simulink model "HydroEye_6DOF_OpenLoop"  (R2024b)
settings: Solver=VariableStepAuto  StartTime=0.0  StopTime=120  RelTol=1e-3
undefined symbols (not defined in the file or in its folder): b, c, CD, cg, CL, Cl, Clp, Clr, Cm, Cmq, Cn, Cnp, Cnr, cp, CY, Earth, mass, WGS84
libraries: simulink_extras x4, aerolibasang x2, shared6dof x1, aerolibatmos2 x1, aerolibadyn x1, aerolibtransform2 x1
settings Model: Creator=01  LastModifiedBy=01
settings OptimizationCC: ReuseModelBlockBuffer=off
settings RTWCC: GPUComputeCapability=3.5

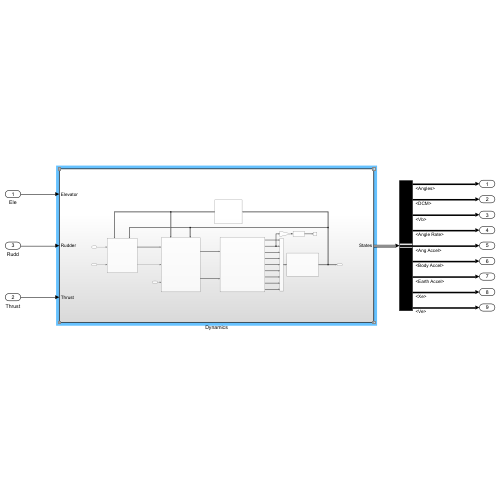
[thumbnail: Simulink's stored preview of the top-level diagram]
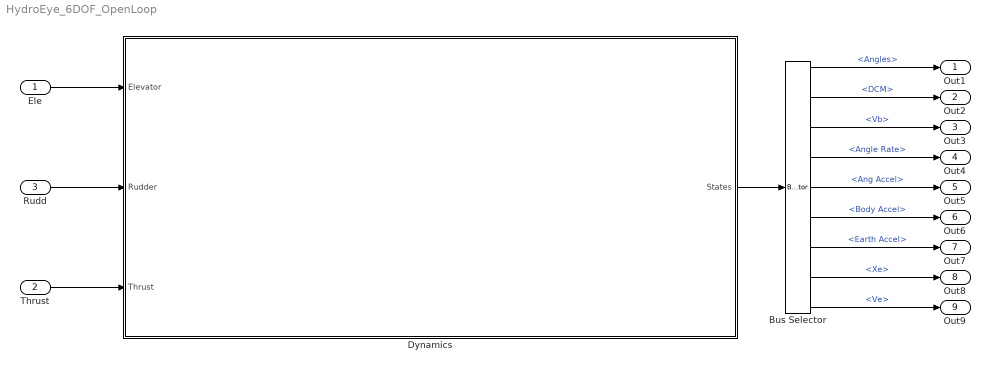
== system HydroEye_6DOF_OpenLoop ==
  Ele : Inport
  Thrust : Inport  Port=2
  Rudd : Inport  Port=3
  Bus Selector : BusSelector  OutputSignals=Raw States.Angles,Raw States.DCM,Raw States.Vb,Raw States.Angle Rate,Raw States.Ang Accel,Raw States.Body Accel,Raw States.Earth Accel,Raw States.Xe,Raw States.Ve
  Dynamics : Subsystem
  Out1 : Outport
  Out2 : Outport  Port=2
  Out3 : Outport  Port=3
  Out4 : Outport  Port=4
  Out5 : Outport  Port=5
  Out6 : Outport  Port=6
  Out7 : Outport  Port=7
  Out8 : Outport  Port=8
  Out9 : Outport  Port=9
  wires:
  Ele/1 -> Dynamics/1(Elevator)
  Thrust/1 -> Dynamics/3(Thrust)
  Dynamics/1(States) -> Bus Selector/1
  Bus Selector/1 -> Out1/1  "<Angles>"
  Bus Selector/2 -> Out2/1  "<DCM>"
  Bus Selector/3 -> Out3/1  "<Vb>"
  Bus Selector/4 -> Out4/1  "<Angle Rate>"
  Bus Selector/5 -> Out5/1  "<Ang Accel>"
  Bus Selector/6 -> Out6/1  "<Body Accel>"
  Bus Selector/7 -> Out7/1  "<Earth Accel>"
  Bus Selector/8 -> Out8/1  "<Xe>"
  Bus Selector/9 -> Out9/1  "<Ve>"
  Rudd/1 -> Dynamics/2(Rudder)

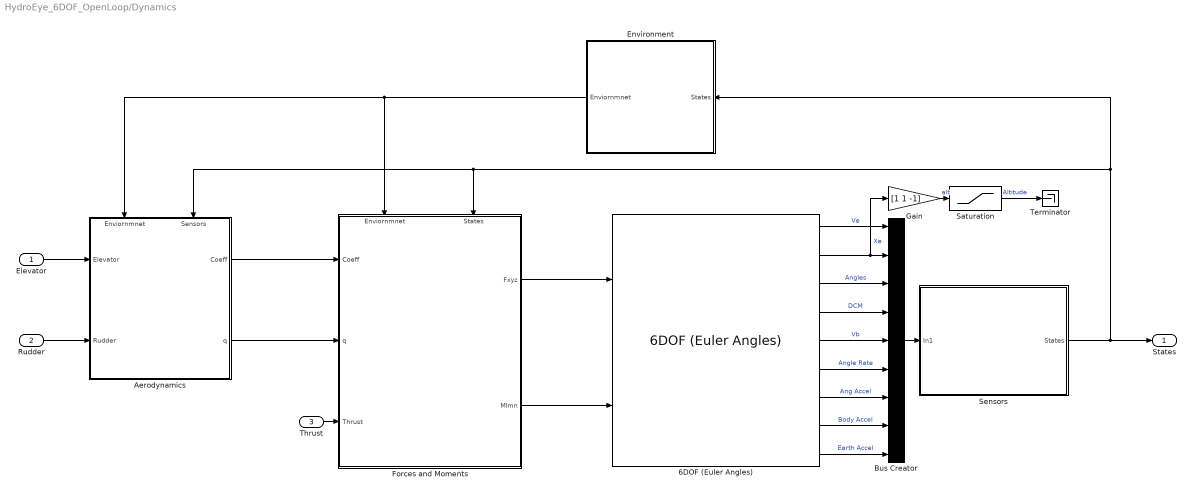
== system HydroEye_6DOF_OpenLoop/Dynamics ==
  Elevator : Inport
  Rudder : Inport  Port=2
  Thrust : Inport  Port=3
  6DOF (Euler Angles) : shared6dof/6DOF (Euler Angles)  units=Metric (MKS)  mtype=Fixed  rep=Euler Angles  xme_0=init.pos  Vm_0=init.v  eul_0=[ 0 deg2rad(2.4) 0 ]  pm_0=[ 0 0 0 ]  mass_0=mass  mass_e=0.5  mass_f=2.0  inertia=I  inertia_e=eye(3)  inertia_f=2*eye(3)  k_quat=1.0  vre_flag=on  abi_flag=on  aMode=aMode  xme_statename=''  Vm_statename=''  eul_statename=''  quat_statename=''  pm_statename=''  mass_statename=''
      settings: LibrarySourceBlock=|
      | aeroblk_lib_HL20/HL20
      | Airframe/6DOF (Euler Angles)
  Aerodynamics : Subsystem
      settings: PortSchema="{\"entries\":[{\"content\":{\"sides\":[{\"content\":{\"connectorIds\":[\"In1\",\"In2\"]},\"type\":\"ConnectorPlacement.EquallySpacedRectSide\",\"uuid\":\"6872a9e6-04cc-43fe-8307-2d3d33caa71d\"},{\"content\":{\"side\":\"RIGHT\"},\"type\":\"ConnectorPlacement.EquallySpacedRectSide\",\"uuid\":\"de5f8d1c-5c0e-46cb-94c5-3e4cce4cf93c\"},{\"content\":{\"connectorIds\":[\"In3\",\"In4\"],\"side\":\"TOP\"},\"type\":\"ConnectorPlacement.EquallySpacedRectSide\",\"uuid\":\"d9dd98e0-8ff1-4387-90e5-0ec057a718ca\"},{\"content\":{\"connectorIds\":[\"Out1\",\"Out2\"],\"side\":\"BOTTOM\"},\"type\":\"ConnectorPlacement.EquallySpacedRectSide\",\"uuid\":\"12421dae-0177-4f1a-9b31-64f8981b692b\"}]},\"type\":\"ConnectorPlacement.EquallySpacedConnector\",\"uuid\":\"9e39648a-6fb6-4479-b0ac-1c0f654141e6\"}],\"packageUris\":[\"http://schema.mathworks.com/mf0/Connector/R2020b\"],\"version\":\"1.0\"}"
  Bus Creator : BusCreator  Inputs=9
  "Environment " : Subsystem
      settings: LibrarySourceBlock=|
      | aeroblk_lib_HL20/HL20
      | Airframe/Environment Models
  Forces and Moments : Subsystem
      settings: PortSchema="{\"entries\":[{\"content\":{\"sides\":[{\"content\":{\"connectorIds\":[\"In1\",\"In2\",\"In3\"]},\"type\":\"ConnectorPlacement.EquallySpacedRectSide\",\"uuid\":\"3fce203a-ae0b-4bce-a87b-30de4173aaf5\"},{\"content\":{\"connectorIds\":[\"Out1\",\"Out2\"],\"side\":\"RIGHT\"},\"type\":\"ConnectorPlacement.EquallySpacedRectSide\",\"uuid\":\"d2fe57eb-25a4-4a3f-81a0-5ad8de127e30\"},{\"content\":{\"connectorIds\":[\"In4\",\"In5\"],\"side\":\"TOP\"},\"type\":\"ConnectorPlacement.EquallySpacedRectSide\",\"uuid\":\"a48e6f39-78f9-49f0-a87f-61fc55168fed\"}]},\"type\":\"ConnectorPlacement.EquallySpacedConnector\",\"uuid\":\"9bf99150-9e27-4a02-9f3a-86824a85a991\"}],\"packageUris\":[\"http://schema.mathworks.com/mf0/Connector/R2020b\"],\"version\":\"1.0\"}"
      settings: LibrarySourceBlock=|
      | aeroblk_lib_HL20/HL20
      | Airframe/Forces and Moments
  Gain : Gain  Gain=[1 1 -1]
  Saturation : Saturate  UpperLimit=inf  LowerLimit=0
  Sensors : Subsystem
  Terminator : Terminator
  States : Outport
  wires:
  6DOF (Euler Angles)/6 -> Bus Creator/6  "Angle Rate"
  6DOF (Euler Angles)/5 -> Bus Creator/5  "Vb"
  Aerodynamics/1(Coeff) -> Forces and Moments/1(Coeff)
  6DOF (Euler Angles)/9 -> Bus Creator/9  "Earth Accel"
  Gain/1 -> Saturation/1  "alt"
  Aerodynamics/2(q) -> Forces and Moments/2(q)
  6DOF (Euler Angles)/1 -> Bus Creator/1  "Ve"
  6DOF (Euler Angles)/3 -> Bus Creator/3  "Angles"
  6DOF (Euler Angles)/7 -> Bus Creator/7  "Ang Accel"
  6DOF (Euler Angles)/4 -> Bus Creator/4  "DCM"
  Bus Creator/1 -> Sensors/1(In1)
  "Environment "/1(Enviornmnet) -> Forces and Moments/4(Enviornmnet), Aerodynamics/1(Enviornmnet)
  Forces and Moments/2(Mlmn) -> 6DOF (Euler Angles)/2
  Forces and Moments/1(Fxyz) -> 6DOF (Euler Angles)/1
  Saturation/1 -> Terminator/1  "Altitude"
  Sensors/1(States) -> "Environment "/1(States), Aerodynamics/2(Sensors), Forces and Moments/5(States), States/1
  6DOF (Euler Angles)/2 -> Gain/1, Bus Creator/2  "Xe"
  6DOF (Euler Angles)/8 -> Bus Creator/8  "Body Accel"
  Elevator/1 -> Aerodynamics/3(Elevator)
  Thrust/1 -> Forces and Moments/3(Thrust)
  Rudder/1 -> Aerodynamics/4(Rudder)

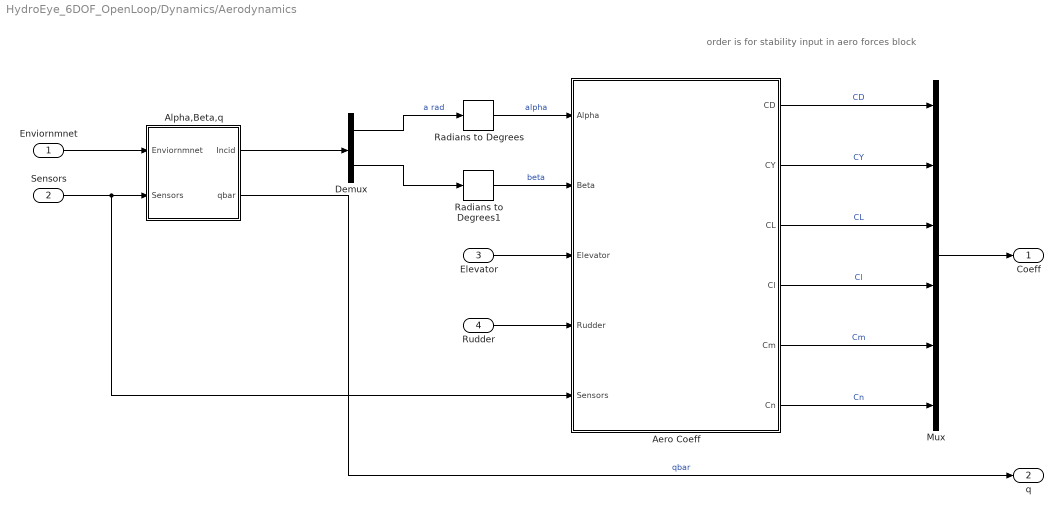
== system HydroEye_6DOF_OpenLoop/Dynamics/Aerodynamics ==
  note: order is for stability input in aero forces block
  Enviornmnet : Inport
  Sensors : Inport  Port=2
  Elevator : Inport  Port=3
  Rudder : Inport  Port=4
  Aero Coeff : Subsystem
  Alpha,Beta,q : Subsystem
      settings: LibrarySourceBlock=|
      | aeroblk_lib_HL20/HL20
      | Airframe/Alpha,Beta,Mach
  Demux : Demux  Outputs=2
  Mux : Mux  Inputs=6
  Radians to Degrees : simulink_extras/Transformations/Radians to Degrees
  Radians to Degrees1 : simulink_extras/Transformations/Radians to Degrees
  Coeff : Outport
  q : Outport  Port=2
  wires:
  Sensors/1 -> Aero Coeff/5(Sensors), Alpha,Beta,q/2(Sensors)
  Enviornmnet/1 -> Alpha,Beta,q/1(Enviornmnet)
  Alpha,Beta,q/2(qbar) -> q/1  "qbar"
  Mux/1 -> Coeff/1
  Alpha,Beta,q/1(Incid) -> Demux/1
  Aero Coeff/1(CD) -> Mux/1  "CD"
  Aero Coeff/2(CY) -> Mux/2  "CY"
  Aero Coeff/3(CL) -> Mux/3  "CL"
  Aero Coeff/4(Cl) -> Mux/4  "Cl"
  Aero Coeff/5(Cm) -> Mux/5  "Cm"
  Aero Coeff/6(Cn) -> Mux/6  "Cn"
  Radians to Degrees/1 -> Aero Coeff/1(Alpha)  "alpha"
  Radians to Degrees1/1 -> Aero Coeff/2(Beta)  "beta"
  Demux/2 -> Radians to Degrees1/1
  Demux/1 -> Radians to Degrees/1  "a rad"
  Elevator/1 -> Aero Coeff/3(Elevator)
  Rudder/1 -> Aero Coeff/4(Rudder)

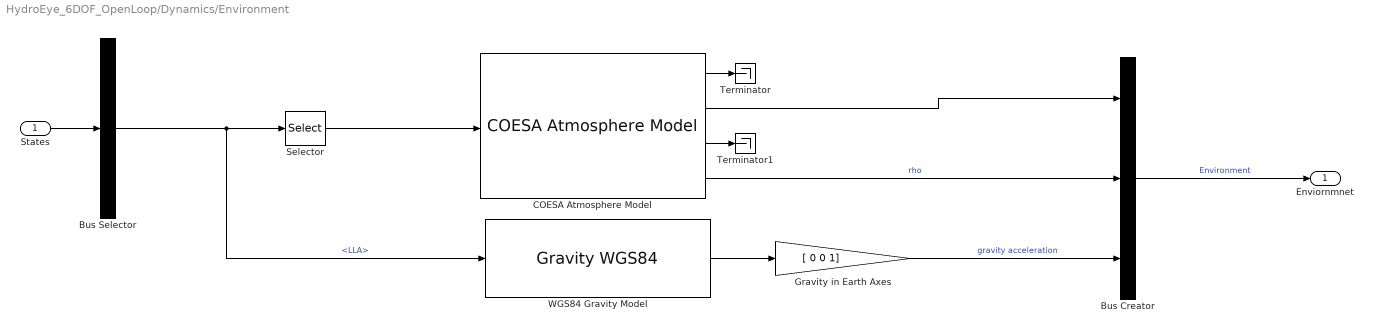
== system HydroEye_6DOF_OpenLoop/Dynamics/Environment  ==
  States : Inport
  Bus Creator : BusCreator  Inputs=3
  Bus Selector : BusSelector  OutputSignals=LLA
  COESA Atmosphere Model : aerolibatmos2/COESA Atmosphere Model  units=Metric (MKS)  spec=1976 COESA-extended U.S. Standard Atmosphere  model=Profile  profile_var=High temperature  profile_percent=10%  profile_alt=5 km (16404 ft)  envelope_var=High temperature  envelope_percent=1%  action=None
      settings: LibrarySourceBlock=|
      | aeroblk_lib_HL20/HL20
      | Airframe/Environment Models/COESA Atmosphere Model
  Gravity in Earth Axes : Gain  Gain=[ 0 0 1]  SaturateOnIntegerOverflow=on  OutDataTypeStr=Inherit: Same as input  ParamDataTypeStr=Inherit: Same as input
  Selector : Selector  InputPortWidth=3  IndexOptions=Index vector (dialog)  Indices=3  OutputSizes=1
  Terminator : Terminator
  Terminator1 : Terminator
  "WGS84 Gravity Model  " : GravityWGS84  action=None
  Enviornmnet : Outport
  wires:
  "WGS84 Gravity Model  "/1 -> Gravity in Earth Axes/1
  COESA Atmosphere Model/1 -> Terminator/1
  COESA Atmosphere Model/3 -> Terminator1/1
  COESA Atmosphere Model/2 -> Bus Creator/1
  COESA Atmosphere Model/4 -> Bus Creator/2  "rho"
  Selector/1 -> COESA Atmosphere Model/1
  Gravity in Earth Axes/1 -> Bus Creator/3  "gravity acceleration"
  States/1 -> Bus Selector/1
  Bus Selector/1 -> "WGS84 Gravity Model  "/1, Selector/1  "<LLA>"
  Bus Creator/1 -> Enviornmnet/1  "Environment"

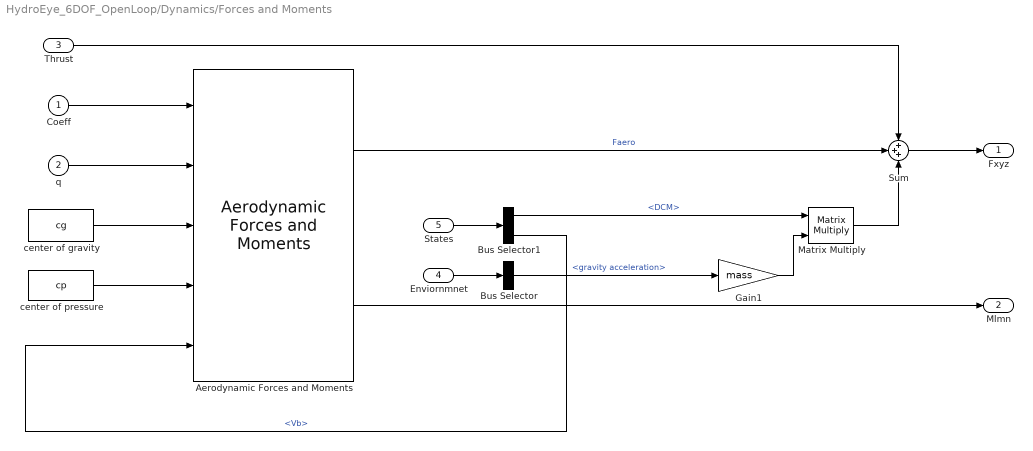
== system HydroEye_6DOF_OpenLoop/Dynamics/Forces and Moments ==
  Coeff : Inport
  q : Inport  Port=2  Unit=Pa
  Thrust : Inport  Port=3
  Enviornmnet : Inport  Port=4
  States : Inport  Port=5
  Aerodynamic Forces and Moments : aerolibadyn/Aerodynamic Forces and Moments   inputAxes=Stability  outputForceAxes=Body  outputMomentAxes=Body  S=Sref  b=b  cbar=c
      settings: LibrarySourceBlock=|
      | aeroblk_lib_HL20/HL20
      | Airframe/Forces and Moments/Aerodynamic
      | Forces and Moments
  Bus Selector : BusSelector  OutputSignals=gravity acceleration
  Bus Selector1 : BusSelector  OutputSignals=Raw States.DCM,Raw States.Vb
  Gain1 : Gain  Gain=mass
  Matrix Multiply : Product  Multiplication=Matrix(*)
  Sum : Sum  Inputs=+++  InputSameDT=on  SaturateOnIntegerOverflow=on  OutDataTypeStr=Inherit: Same as first input
  center of gravity : Constant  Value=cg
  center of pressure : Constant  Value=cp
  Fxyz : Outport
  Mlmn : Outport  Port=2
  wires:
  Coeff/1 -> Aerodynamic Forces and Moments/1
  q/1 -> Aerodynamic Forces and Moments/2
  Sum/1 -> Fxyz/1
  center of gravity/1 -> Aerodynamic Forces and Moments/3
  center of pressure/1 -> Aerodynamic Forces and Moments/4
  Enviornmnet/1 -> Bus Selector/1
  States/1 -> Bus Selector1/1
  Matrix Multiply/1 -> Sum/3
  Bus Selector/1 -> Gain1/1  "<gravity acceleration>"
  Gain1/1 -> Matrix Multiply/2
  Bus Selector1/1 -> Matrix Multiply/1  "<DCM>"
  Thrust/1 -> Sum/1
  Aerodynamic Forces and Moments/1 -> Sum/2  "Faero"
  Aerodynamic Forces and Moments/2 -> Mlmn/1
  Bus Selector1/2 -> Aerodynamic Forces and Moments/5  "<Vb>"

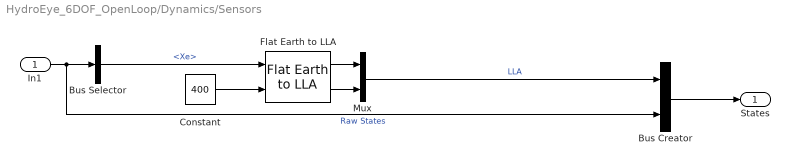
== system HydroEye_6DOF_OpenLoop/Dynamics/Sensors ==
  In1 : Inport
  Bus Creator : BusCreator  Inputs=2
  Bus Selector : BusSelector  OutputSignals=Xe
  Constant : Constant  Value=400
  Flat Earth to LLA : aerolibtransform2/Flat Earth to LLA  units=Metric (MKS)  ptype=Earth (WGS84)  F=1/298.257223563  R=6378137  refPosPort=off  LL0=[ 24 46 ]  psi=0
  Mux : Mux  Inputs=2
  States : Outport
  wires:
  In1/1 -> Bus Creator/2, Bus Selector/1  "Raw States"
  Bus Selector/1 -> Flat Earth to LLA/1  "<Xe>"
  Flat Earth to LLA/2 -> Mux/2
  Flat Earth to LLA/1 -> Mux/1
  Mux/1 -> Bus Creator/1  "LLA"
  Bus Creator/1 -> States/1
  Constant/1 -> Flat Earth to LLA/2

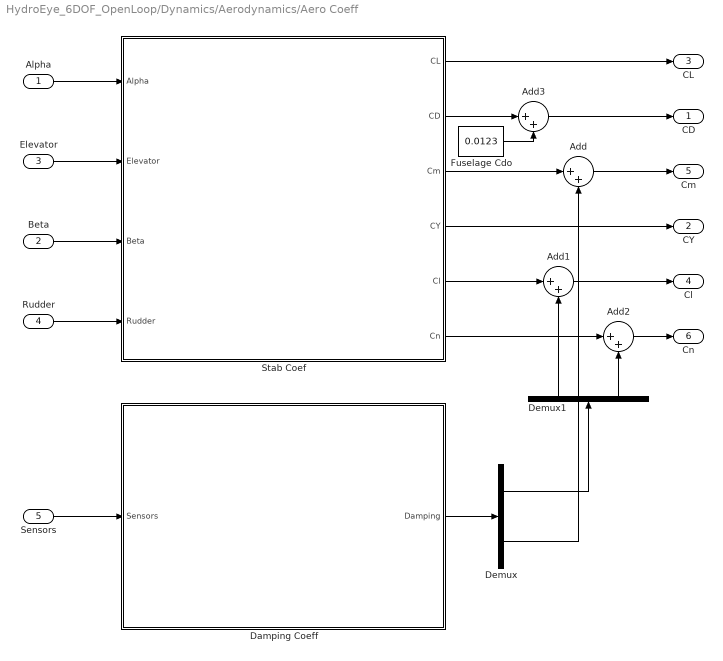
== system HydroEye_6DOF_OpenLoop/Dynamics/Aerodynamics/Aero Coeff ==
  Alpha : Inport
  Beta : Inport  Port=2
  Elevator : Inport  Port=3
  Rudder : Inport  Port=4
  Sensors : Inport  Port=5
  Add{,1..3} (4 alike) : Sum  Inputs=|++
  Damping Coeff : Subsystem
  Demux : Demux  Outputs=2
  Demux1 : Demux  Outputs=2
  Fuselage Cdo : Constant  Value=0.0123
  Stab Coef : Subsystem
  CD : Outport
  CY : Outport  Port=2
  CL : Outport  Port=3
  Cl : Outport  Port=4
  Cm : Outport  Port=5
  Cn : Outport  Port=6
  wires:
  Alpha/1 -> Stab Coef/1(Alpha)
  Elevator/1 -> Stab Coef/2(Elevator)
  Beta/1 -> Stab Coef/3(Beta)
  Rudder/1 -> Stab Coef/4(Rudder)
  Stab Coef/1(CL) -> CL/1
  Stab Coef/4(CY) -> CY/1
  Sensors/1 -> Damping Coeff/1(Sensors)
  Damping Coeff/1(Damping) -> Demux/1
  Stab Coef/3(Cm) -> Add/1
  Add/1 -> Cm/1
  Demux/2 -> Add/2
  Stab Coef/5(Cl) -> Add1/1
  Add1/1 -> Cl/1
  Add2/1 -> Cn/1
  Stab Coef/6(Cn) -> Add2/1
  Demux/1 -> Demux1/1
  Demux1/2 -> Add2/2
  Demux1/1 -> Add1/2
  Stab Coef/2(CD) -> Add3/1
  Add3/1 -> CD/1
  Fuselage Cdo/1 -> Add3/2

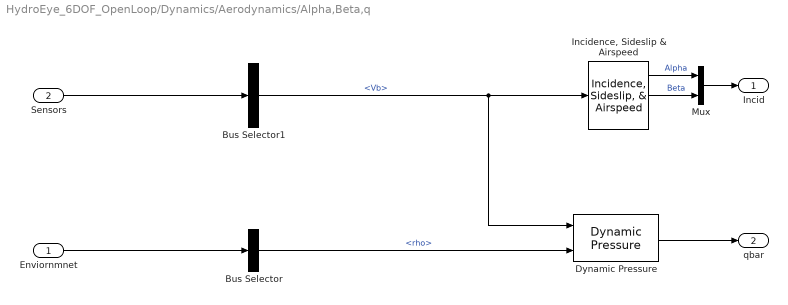
== system HydroEye_6DOF_OpenLoop/Dynamics/Aerodynamics/Alpha,Beta,q ==
  Enviornmnet : Inport
  Sensors : Inport  Port=2
  Bus Selector : BusSelector  OutputSignals=rho
  Bus Selector1 : BusSelector  OutputSignals=Raw States.Vb
  Dynamic Pressure : aerolibasang/Dynamic Pressure
      settings: LibrarySourceBlock=|
      | aeroblk_lib_HL20/HL20
      | Airframe/Alpha,Beta,Mach/Dynamic Pressure
  "Incidence, Sideslip & Airspeed" : aerolibasang/Incidence, Sideslip, & Airspeed
      settings: LibrarySourceBlock=|
      | aeroblk_lib_HL20/HL20
      | Airframe/Alpha,Beta,Mach/Incidence, Sideslip
      | & Airspeed
  Mux : Mux  Inputs=2
  Incid : Outport  Unit=rad  VectorParamsAs1DForOutWhenUnconnected=off
  qbar : Outport  Port=2  Unit=Pa  InitialOutput=0  VectorParamsAs1DForOutWhenUnconnected=off
  wires:
  "Incidence, Sideslip & Airspeed"/1 -> Mux/1  "Alpha"
  Mux/1 -> Incid/1
  "Incidence, Sideslip & Airspeed"/2 -> Mux/2  "Beta"
  Dynamic Pressure/1 -> qbar/1
  Enviornmnet/1 -> Bus Selector/1
  Bus Selector/1 -> Dynamic Pressure/2  "<rho>"
  Sensors/1 -> Bus Selector1/1
  Bus Selector1/1 -> "Incidence, Sideslip & Airspeed"/1, Dynamic Pressure/1  "<Vb>"

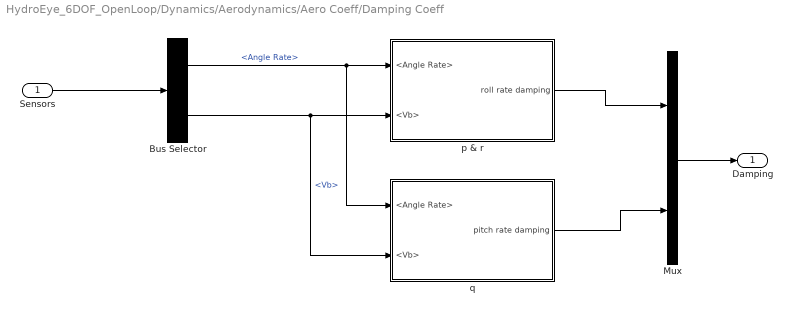
== system HydroEye_6DOF_OpenLoop/Dynamics/Aerodynamics/Aero Coeff/Damping Coeff ==
  Sensors : Inport
  Bus Selector : BusSelector  OutputSignals=Raw States.Angle Rate,Raw States.Vb
  Mux : Mux  Inputs=2
  p & r : Subsystem
  q : Subsystem
  Damping : Outport
  wires:
  Sensors/1 -> Bus Selector/1
  q/1(pitch rate damping) -> Mux/2
  Mux/1 -> Damping/1
  p & r/1(roll rate damping) -> Mux/1
  Bus Selector/1 -> q/1(<Angle Rate>), p & r/1(<Angle Rate>)  "<Angle Rate>"
  Bus Selector/2 -> q/2(<Vb>), p & r/2(<Vb>)  "<Vb>"

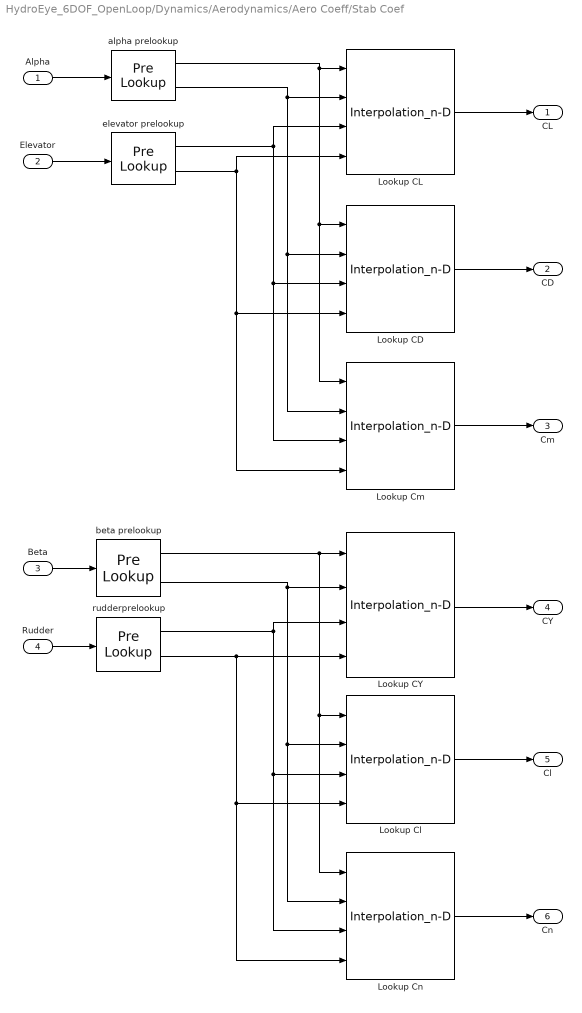
== system HydroEye_6DOF_OpenLoop/Dynamics/Aerodynamics/Aero Coeff/Stab Coef ==
  Alpha : Inport
  Elevator : Inport  Port=2
  Beta : Inport  Port=3
  Rudder : Inport  Port=4
  Lookup CD : Interpolation_n-D  Table=CD  InternalRulePriority=Speed
  Lookup CL : Interpolation_n-D  Table=CL  InternalRulePriority=Speed
  Lookup CY : Interpolation_n-D  Table=CY  InternalRulePriority=Speed
  Lookup Cl : Interpolation_n-D  Table=Cl  InternalRulePriority=Speed
  Lookup Cm : Interpolation_n-D  Table=Cm  InternalRulePriority=Speed
  Lookup Cn : Interpolation_n-D  Table=Cn  InternalRulePriority=Speed
  alpha prelookup : PreLookup  BreakpointsData=alpha  BeginIndexSearchUsingPreviousIndexResult=on  ExtrapMethod=Linear
  beta prelookup : PreLookup  BreakpointsData=beta  ExtrapMethod=Linear
  elevator prelookup : PreLookup  BreakpointsData=elevator  ExtrapMethod=Linear
  rudderprelookup : PreLookup  BreakpointsData=rudder  ExtrapMethod=Linear
  CL : Outport
  CD : Outport  Port=2
  Cm : Outport  Port=3
  CY : Outport  Port=4
  Cl : Outport  Port=5
  Cn : Outport  Port=6
  wires:
  beta prelookup/2 -> Lookup Cn/2, Lookup Cl/2, Lookup CY/2
  rudderprelookup/2 -> Lookup Cn/4, Lookup Cl/4, Lookup CY/4
  alpha prelookup/1 -> Lookup Cm/1, Lookup CD/1, Lookup CL/1
  beta prelookup/1 -> Lookup Cn/1, Lookup Cl/1, Lookup CY/1
  elevator prelookup/1 -> Lookup CL/3, Lookup Cm/3, Lookup CD/3
  Lookup Cn/1 -> Cn/1
  Alpha/1 -> alpha prelookup/1
  alpha prelookup/2 -> Lookup Cm/2, Lookup CD/2, Lookup CL/2
  elevator prelookup/2 -> Lookup Cm/4, Lookup CD/4, Lookup CL/4
  Lookup CL/1 -> CL/1
  Rudder/1 -> rudderprelookup/1
  Beta/1 -> beta prelookup/1
  rudderprelookup/1 -> Lookup CY/3, Lookup Cn/3, Lookup Cl/3
  Lookup Cm/1 -> Cm/1
  Elevator/1 -> elevator prelookup/1
  Lookup CY/1 -> CY/1
  Lookup Cl/1 -> Cl/1
  Lookup CD/1 -> CD/1

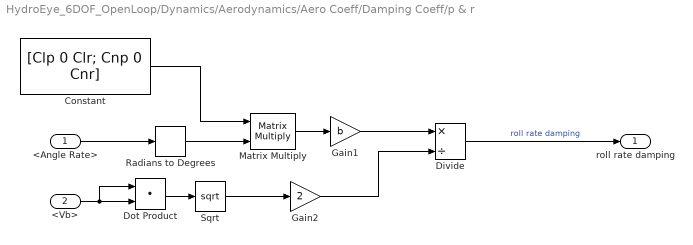
== system HydroEye_6DOF_OpenLoop/Dynamics/Aerodynamics/Aero Coeff/Damping Coeff/p & r ==
  <Angle Rate> : Inport
  <Vb> : Inport  Port=2
  Constant : Constant  Value=[Clp 0 Clr; Cnp 0 Cnr]
  Divide : Product  Inputs=*/
  Dot Product : DotProduct  OutDataTypeStr=Inherit: Inherit via internal rule
  Gain1 : Gain  Gain=b
  Gain2 : Gain  Gain=2
  Matrix Multiply : Product  Multiplication=Matrix(*)
  Radians to Degrees : simulink_extras/Transformations/Radians to Degrees
  Sqrt : Sqrt
  roll rate damping : Outport
  wires:
  Gain2/1 -> Divide/2
  Matrix Multiply/1 -> Gain1/1
  Gain1/1 -> Divide/1
  Divide/1 -> roll rate damping/1  "roll rate damping"
  Constant/1 -> Matrix Multiply/1
  <Vb>/1 -> Dot Product/1, Dot Product/2
  Dot Product/1 -> Sqrt/1
  Sqrt/1 -> Gain2/1
  <Angle Rate>/1 -> Radians to Degrees/1
  Radians to Degrees/1 -> Matrix Multiply/2

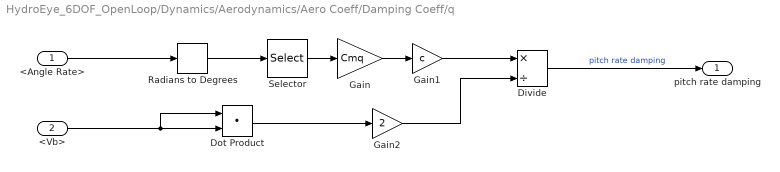
== system HydroEye_6DOF_OpenLoop/Dynamics/Aerodynamics/Aero Coeff/Damping Coeff/q ==
  <Angle Rate> : Inport
  <Vb> : Inport  Port=2
  Divide : Product  Inputs=*/
  Dot Product : DotProduct  OutDataTypeStr=Inherit: Inherit via internal rule
  Gain : Gain  Gain=Cmq
  Gain1 : Gain  Gain=c
  Gain2 : Gain  Gain=2
  Radians to Degrees : simulink_extras/Transformations/Radians to Degrees
  Selector : Selector  InputPortWidth=3  IndexOptions=Index vector (dialog)  Indices=2  OutputSizes=1
  pitch rate damping : Outport
  wires:
  Selector/1 -> Gain/1
  Gain2/1 -> Divide/2
  Gain/1 -> Gain1/1
  Gain1/1 -> Divide/1
  Divide/1 -> pitch rate damping/1  "pitch rate damping"
  <Vb>/1 -> Dot Product/1, Dot Product/2
  Dot Product/1 -> Gain2/1
  <Angle Rate>/1 -> Radians to Degrees/1
  Radians to Degrees/1 -> Selector/1
